simulink model "pt2s_TestBed1_org"  (Simulink 10.0)
settings: Solver=FixedStepDiscrete  StartTime=0.0  StopTime=1  FixedStep=1  RelTol=1e-3  EnableMultiTasking=on
undefined symbols (not defined in the file): MWS
libraries: Lib_Thermo_PT2S_TMATS x1
settings Model: Creator=jwchapm2  LastModifiedBy=annonymous
settings DataIOCC: LimitDataPoints=on
settings OptimizationCC: ExpressionDepthLimit=2147483647
settings DebuggingCC: SolverPrmCheckMsg=warning  StateNameClashWarn=warning
settings GRTTargetCC: GeneratePreprocessorConditionals=Disable all  CombineOutputUpdateFcns=on  GRTInterface=off
settings ConfigComp: CovExternalEMLEnable=off

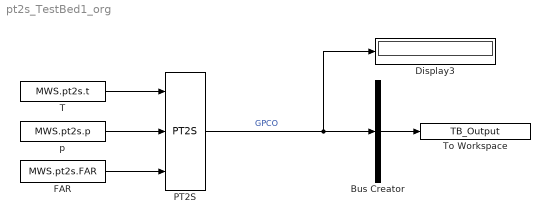
== system pt2s_TestBed1_org ==
  Bus Creator : BusCreator  Inputs=1
  Display3 : Display
  FAR : Constant  Value=MWS.pt2s.FAR
  PT2S : Lib_Thermo_PT2S_TMATS/PT2S
  T : Constant  Value=MWS.pt2s.t
  To Workspace : ToWorkspace  VariableName=TB_Output  SampleTime=-1
  p : Constant  Value=MWS.pt2s.p
  wires:
  FAR/1 -> PT2S/3
  T/1 -> PT2S/1
  PT2S/1 -> Display3/1, Bus Creator/1  "GPCO"
  Bus Creator/1 -> To Workspace/1
  p/1 -> PT2S/2
